simulink model "Two_mass_stifness_system"  (R2018b)
settings: Solver=ode3  StartTime=0.0  StopTime=2  FixedStep=1e-5  RelTol=1e-3  EnableMultiTasking=on
values from neighbouring files (symbols this model uses):
  c = GJp/l    (= 0.0104)    [params.m]
  ce = (Un - In*R)/wn    (= 0.301701587302)    [params.m]
  cm = Mn/In    (= 0.212068965517)    [params.m]
  Jadd = Jm/10    (= 5.9e-06)    [params.m]
  Jm = 0.59*10^(-4)    (= 5.9e-05)    [params.m]
  k_ampl = 1    [params.m]
  kp = 1    [params.m]
  Mn = 0.123    [params.m]
  R = 25.8    [params.m]
settings Model: Creator=user  LastModifiedBy=user
settings DataIOCC: SaveFormat=Array
settings OptimizationCC: DefaultParameterBehavior=Inlined  BufferReuse=off  LifeSpan=inf
settings DebuggingCC: UnderspecifiedInitializationDetection=Classic  MergeDetectMultiDrivingBlocksExec=none  SolverPrmCheckMsg=warning  InitInArrayFormatMsg=none  SFUnexpectedBacktrackingDiag=warning  SFNoUnconditionalDefaultTransitionDiag=warning  SFExecutionAtInitializationDiag=none
settings HardwareCC: ProdBitPerPointer=32  ProdBitPerSizeT=32  ProdBitPerPtrDiffT=32  ProdLargestAtomicFloat=None  ProdIntDivRoundTo=Undefined  ProdEndianess=Unspecified  ProdWordSize=32  ProdHWDeviceType=32-bit Generic
settings ModelReferenceCC: PropagateSignalLabelsOutOfModel=off
settings SFSimCC: SimUseLocalCustomCode=off
settings RTWCC: RTWUseLocalCustomCode=off
settings CodeAppCC: StateflowObjectComments=on
settings GRTTargetCC: TargetLangStandard=C89/C90 (ANSI)  GeneratePreprocessorConditionals=Disable all
settings ConfigComp: CovMetricSettings=dw  CovHtmlReporting=on  CovSaveCumulativeToWorkspaceVar=on  CovSaveSingleToWorkspaceVar=on  CovExternalEMLEnable=off

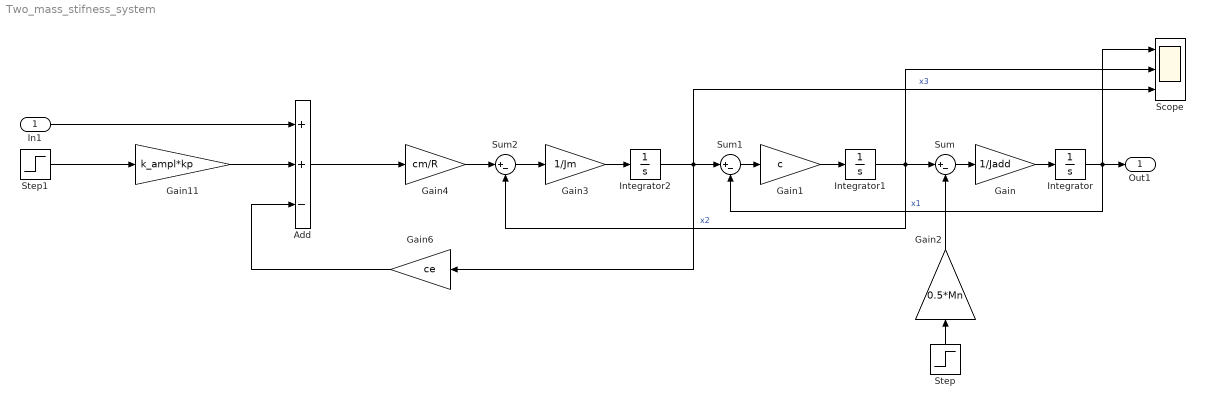
== system Two_mass_stifness_system ==
  In1 : Inport
  Add : Sum  Inputs=++-
  Gain : Gain  Gain=1/Jadd
  Gain1 : Gain  Gain=c
  Gain11 : Gain  Gain=k_ampl*kp
  Gain2 : Gain  Gain=0.5*Mn
  Gain3 : Gain  Gain=1/Jm
  Gain4 : Gain  Gain=cm/R
  Gain6 : Gain  Gain=ce
  Integrator : Integrator
  Integrator1 : Integrator
  Integrator2 : Integrator
  Scope : Scope  NumInputPorts=3
  Step : Step  Time=0  SampleTime=0
  Step1 : Step  Time=0  SampleTime=0
  Sum : Sum  Inputs=|+-
  Sum1 : Sum  Inputs=|+-
  Sum2 : Sum  Inputs=|+-
  Out1 : Outport
  wires:
  Sum/1 -> Gain/1
  Gain/1 -> Integrator/1
  Gain1/1 -> Integrator1/1
  Integrator1/1 -> Sum2/2, Scope/2, Sum/1  "x2"
  Sum1/1 -> Gain1/1
  Integrator/1 -> Sum1/2, Scope/1, Out1/1  "x1"
  Gain3/1 -> Integrator2/1
  Integrator2/1 -> Gain6/1, Scope/3, Sum1/1  "x3"
  Sum2/1 -> Gain3/1
  Gain4/1 -> Sum2/1
  Gain6/1 -> Add/3
  Step/1 -> Gain2/1
  Add/1 -> Gain4/1
  In1/1 -> Add/1
  Gain2/1 -> Sum/2
  Step1/1 -> Gain11/1
  Gain11/1 -> Add/2
